simulink model "digitalfilterdesign_tut"  (Simulink 5.0)
settings: Solver=FixedStepDiscrete  StartTime=0.0  StopTime=2  RelTol=1e-3
libraries: dsparch4 x2, dspsrcs4 x2, simulink x1, dspsnks4 x1
settings Model: Creator=ckamachi  LastModifiedBy=ckamachi  BooleanDataType=off  ProdHWWordLengths=8,32,16,32

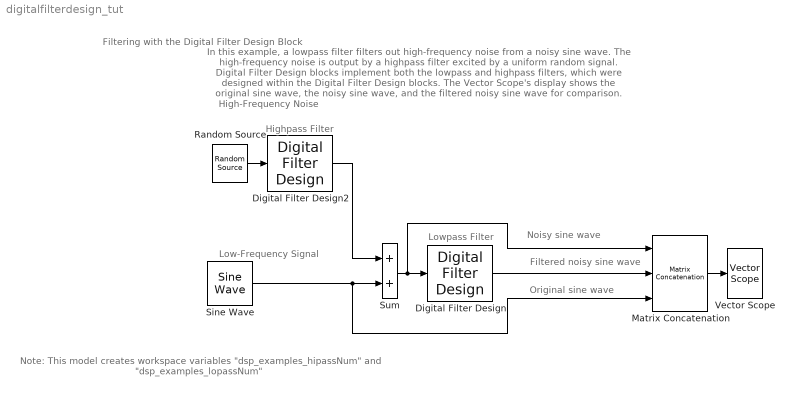
== system digitalfilterdesign_tut ==
  note: High-Frequency Noise
  note: Low-Frequency Signal
  note: Lowpass Filter
  note: Highpass Filter
  note: Noisy sine wave
  note: Filtered noisy sine wave
  note: Original sine wave
  note: Filtering with the
      | Digital Filter Design Block
  note: In this example, a lowpass filter filters out high-frequency
      | noise from a noisy sine wave.  The high-frequency noise is
      | output by a highpass filter excited by a uniform random signal.
      |
      | Digital Filter Design blocks implement both the lowpass and highpass
      | filters, which were designed within the Digital Filter Design blocks.
      | The Vector Scope's display shows the original sine wave,
      | the noisy sine wave, and the filtered noisy sine wave for comparison.
  note: Note: This model creates workspace variables "dsp_examples_hipassNum" and "dsp_examples_lopassNum"
  Digital Filter Design : dsparch4/Digital Filter Design
  Digital Filter Design2 : dsparch4/Digital Filter Design
  Matrix Concatenation : simulink/Math Operations/Matrix Concatenation  numInports=3  catMethod=Horizontal
  Random Source : dspsrcs4/Random Source  SrcType=Uniform  NormMethod=Ziggurat  CltLength=12  Min=0  Max=4  Mean=0  Var=1  RepMode=Not repeatable  Seed=1  Inherit=off  SampMode=Discrete  SampTime=1/1000  SampFrame=50  DataType=Double  OutComplex=Real
  Sine Wave : dspsrcs4/Sine Wave  Amplitude=1  Frequency=75  Phase=0  SampleMode=Discrete  OutComplex=Real  CompMethod=Trigonometric fcn  TableSize=Speed  SampleTime=1/1000  SamplesPerFrame=50  dataType=double  wordLen=16  udDataType=sfix(16)  fracBitsMode=Best precision  numFracBits=14  ResetState=Restart at time zero
  Sum : Sum  SaturateOnIntegerOverflow=on  InputSameDT=on
  Vector Scope : dspsnks4/Vector Scope  ScopeProperties=on  Domain=Time  HorizSpan=1  DisplayProperties=off  AxisGrid=on  Memory=off  FrameNumber=on  AxisLegend=on  AxisZoom=off  OpenScopeAtSimStart=on  OpenScopeImmediately=off  FigPos=[386 364 548 328]  AxisProperties=off  XUnits=Hertz  XRange=[0...Fs/2]  InheritXIncr=on  XIncr=1  XLabel=Time  YUnits=dB  YLabel=Amplitude  LineProperties=off  LineStyles=-||None  LineMarkers=None|diamond|*  LineColors=|[1 0 0]|[0 0 1]
      settings: YMin=-10  YMax=10
  wires:
  Random Source/1 -> Digital Filter Design2/1
  Sine Wave/1 -> Sum/2, Matrix Concatenation/3
  Sum/1 -> Matrix Concatenation/1, Digital Filter Design/1
  Matrix Concatenation/1 -> Vector Scope/1
  Digital Filter Design/1 -> Matrix Concatenation/2
  Digital Filter Design2/1 -> Sum/1
